simulink model "SemiOffline_DataImport"  (R2019a)
settings: Solver=FixedStepDiscrete  StartTime=0.0  StopTime=2*sim_time  FixedStep=1/fs  MaxStep=1/fs  RelTol=1e-3
undefined symbols (not defined in the file): fs
settings Model: PacingRate=100  Creator=rcord  LastModifiedBy=rcord
settings SolverCC: ZeroCrossControl=DisableAll
settings DataIOCC: ExternalInput=[t, ecg, x, y, z]  LoadExternalInput=on  LoggingIntervals=[-inf,inf]

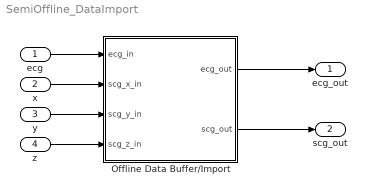
== system SemiOffline_DataImport ==
  ecg : Inport  SampleTime=1/fs
  x : Inport  Port=2  SampleTime=1/fs
  y : Inport  Port=3  SampleTime=1/fs
  z : Inport  Port=4  SampleTime=1/fs
  Offline Data Buffer/Import : Subsystem  mask{param_frame_size_sec=12}
      mask prompts: param_frame_size_sec "Frame Size (in seconds)"
      mask init:
      | assignin('base','param_frame_size_sec',param_frame_size_sec)
      mask DialogControl DescGroupVar Prompt: Data Import Buffer
      mask DialogControl DescTextVar Prompt: The buffer size will specify the length of the jumping "frame" or "window". Subsequent analysis will be performed on each of these windows in succession.
  ecg_out : Outport
  scg_out : Outport  Port=2
  wires:
  ecg/1 -> Offline Data Buffer/Import/1(ecg_in)
  x/1 -> Offline Data Buffer/Import/2(scg_x_in)
  y/1 -> Offline Data Buffer/Import/3(scg_y_in)
  z/1 -> Offline Data Buffer/Import/4(scg_z_in)
  Offline Data Buffer/Import/1(ecg_out) -> ecg_out/1
  Offline Data Buffer/Import/2(scg_out) -> scg_out/1

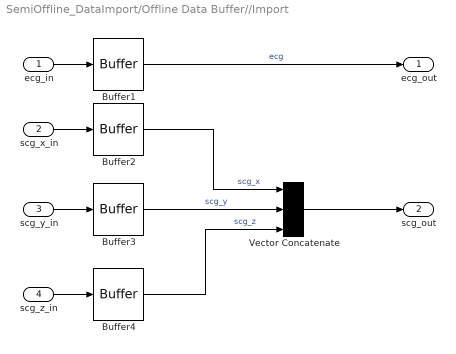
== system SemiOffline_DataImport/Offline Data Buffer//Import ==
  ecg_in : Inport
  scg_x_in : Inport  Port=2
  scg_y_in : Inport  Port=3
  scg_z_in : Inport  Port=4
  Buffer{1..4} (4 alike) : Buffer  N=param_frame_size_sec*fs  OutputFrames=off
  Vector Concatenate : Concatenate  NumInputs=3  Mode=Multidimensional array  ConcatenateDimension=2
  ecg_out : Outport
  scg_out : Outport  Port=2
  wires:
  ecg_in/1 -> Buffer1/1
  Buffer4/1 -> Vector Concatenate/3  "scg_z"
  Buffer2/1 -> Vector Concatenate/1  "scg_x"
  scg_x_in/1 -> Buffer2/1
  Vector Concatenate/1 -> scg_out/1
  Buffer1/1 -> ecg_out/1  "ecg"
  Buffer3/1 -> Vector Concatenate/2  "scg_y"
  scg_z_in/1 -> Buffer4/1
  scg_y_in/1 -> Buffer3/1
